simulink model "test_system_2016a"  (R2018b)
settings: Solver=VariableStepAuto  StartTime=0.0  StopTime=80  FixedStep=0.02  RelTol=1e-3  EnableMultiTasking=on
values from neighbouring files (symbols this model uses):
  c0 = g0    [init_transfers_knut.m]
  D = 50    [init_transfers_knut.m]
  FD = -X22*Y21    [init_transfers_knut.m]
  FD_f = 1    [init_transfers_knut.m]
  g0 = q0    [init_transfers_knut.m]
  H = 3.5    [init_transfers_knut.m]
  H2 = 9.6    [init_transfers_knut.m]
  hs = 1    [init_transfers_knut.m]
  K11 = 2*pi*f0*S_base/M1*bd1*(1-bd1*X22(1,1))    [init_transfers_knut.m]
  K12 = 2*pi*f0*S_base/M1*bd1*bd2*X22(1,2)    [init_transfers_knut.m]
  K13 = S_base/M1*bd1*X22(1,3)    [init_transfers_knut.m]
  K21 = 2*pi*f0*S_base/M2*bd1*bd2*X22(2,1)    [init_transfers_knut.m]
  K22 = 2*pi*f0*S_base/M2*bd2*(1-bd2*X22(2,2))    [init_transfers_knut.m]
  K23 = S_base/M2*bd2*X22(2,3)    [init_transfers_knut.m]
  Kd = 0.5    [init_transfers_knut.m]
  Kd2 = 0.1    [init_transfers_knut.m]
  Kp = 10    [init_transfers_knut.m]
  Pm0 = 0.8    [init_transfers_knut.m]
  q0 = (Pm0+(At*qnl))/(At-(w0*Dt))    [init_transfers_knut.m]
  R = 0.08    [init_transfers_knut.m]
  R2 = R    (= 0.08)    [init_transfers_knut.m]
  Td = 0    [init_transfers_knut.m]
  Tf = 0.05    [init_transfers_knut.m]
  Ti = 9.1    [init_transfers_knut.m]
  w0 = 0    [init_transfers_knut.m]
  w_ref = w0+g0*R    [init_transfers_knut.m]
undefined symbols (not defined in the file or in its folder): At, Dt, Gmax, Gmin, qnl, r, Tg, Tr, Tw
settings Model: Creator=sigurdj  LastModifiedBy=sigurd
settings DataIOCC: LimitDataPoints=on  SaveFormat=Array
settings OptimizationCC: LifeSpan=inf
settings DebuggingCC: SolverPrmCheckMsg=warning  SFUnexpectedBacktrackingDiag=warning  SFNoUnconditionalDefaultTransitionDiag=warning
settings HardwareCC: ProdBitPerPointer=32  ProdBitPerSizeT=32  ProdBitPerPtrDiffT=32  ProdLargestAtomicFloat=None  ProdIntDivRoundTo=Undefined  ProdEndianess=Unspecified  ProdWordSize=32  ProdHWDeviceType=32-bit Generic
settings ModelReferenceCC: PropagateSignalLabelsOutOfModel=off
settings SFSimCC: SimUseLocalCustomCode=off
settings RTWCC: RTWUseLocalCustomCode=off
settings CodeAppCC: StateflowObjectComments=on
settings GRTTargetCC: TargetLangStandard=C89/C90 (ANSI)  GeneratePreprocessorConditionals=Disable all
settings ConfigComp: CovMetricSettings=dw  CovHtmlReporting=on  CovSaveCumulativeToWorkspaceVar=on  CovSaveSingleToWorkspaceVar=on  CovExternalEMLEnable=off  CovSFcnEnable=off

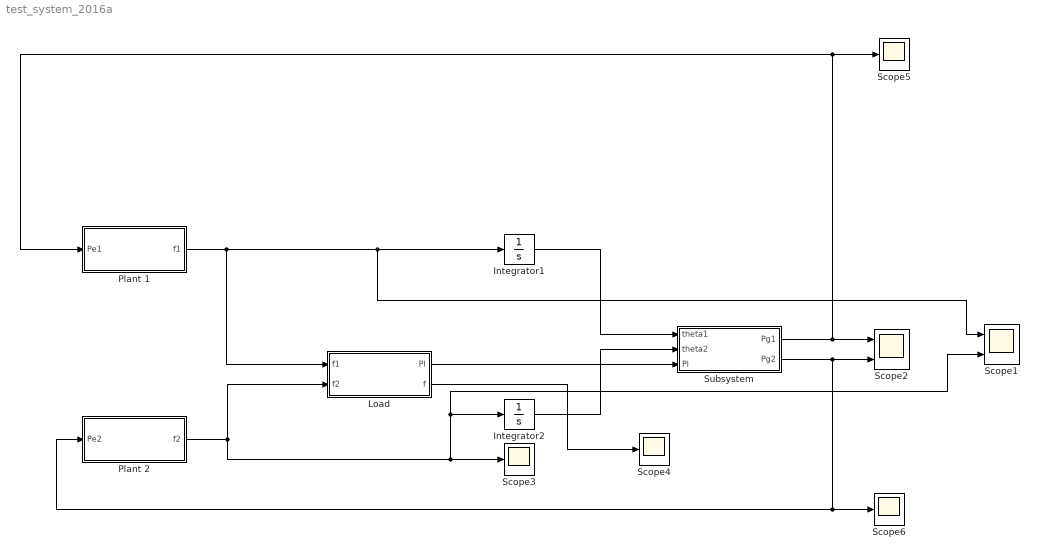
== system test_system_2016a ==
  Integrator1 : Integrator
  Integrator2 : Integrator
  Load : Subsystem
  Plant 1 : Subsystem
  Plant 2 : Subsystem
  Scope1 : Scope  NumInputPorts=2
  Scope2 : Scope  NumInputPorts=2
  Scope{3..6} (4 alike) : Scope
  Subsystem : Subsystem
  wires:
  Integrator2/1 -> Subsystem/2(theta2)
  Subsystem/2(Pg2) -> Scope2/2, Plant 2/1(Pe2), Scope6/1
  Plant 1/1(f1) -> Integrator1/1, Scope1/1, Load/1(f1)
  Plant 2/1(f2) -> Load/2(f2), Integrator2/1, Scope1/2, Scope3/1
  Integrator1/1 -> Subsystem/1(theta1)
  Subsystem/1(Pg1) -> Plant 1/1(Pe1), Scope5/1, Scope2/1
  Load/1(Pl) -> Subsystem/3(Pl)
  Load/2(f) -> Scope4/1

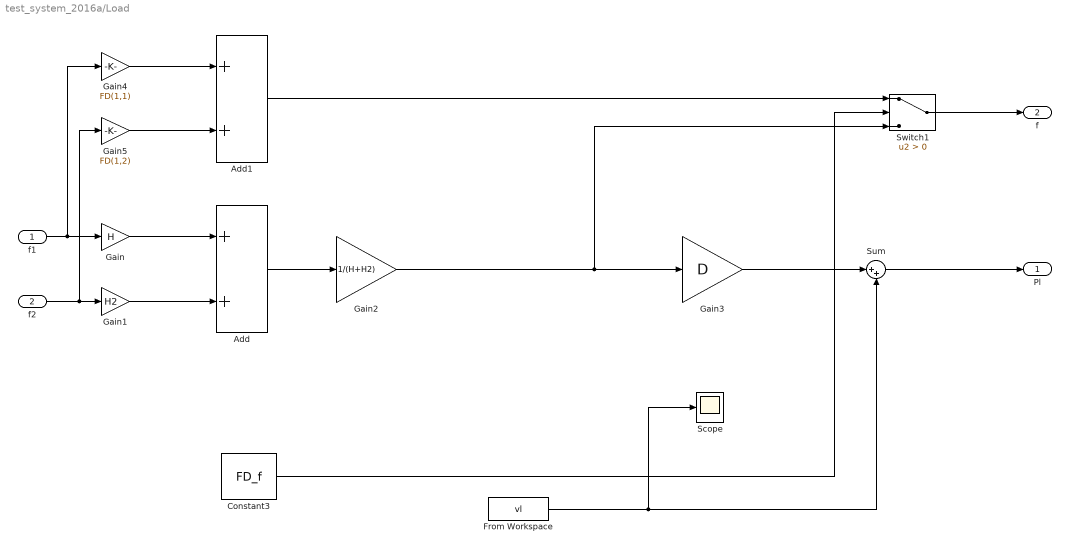
== system test_system_2016a/Load ==
  f1 : Inport
  f2 : Inport  Port=2
  Add : Sum
  Add1 : Sum
  Constant3 : Constant  Value=FD_f
  From Workspace : FromWorkspace  VariableName=vl  SampleTime=0
  Gain : Gain  Gain=H
  Gain1 : Gain  Gain=H2
  Gain2 : Gain  Gain=1/(H+H2)
  Gain3 : Gain  Gain=D
  Gain4 : Gain  Gain=FD(1,1)
  Gain5 : Gain  Gain=FD(1,2)
  Scope : Scope
  Sum : Sum  Inputs=|++
  Switch1 : Switch  Criteria=u2 > Threshold
  Pl : Outport
  f : Outport  Port=2
  wires:
  f2/1 -> Gain5/1, Gain1/1
  Gain/1 -> Add/1
  Gain1/1 -> Add/2
  Add/1 -> Gain2/1
  Sum/1 -> Pl/1
  From Workspace/1 -> Scope/1, Sum/2
  Gain2/1 -> Switch1/3, Gain3/1
  Gain4/1 -> Add1/1
  Gain5/1 -> Add1/2
  Add1/1 -> Switch1/1
  f1/1 -> Gain4/1, Gain/1
  Constant3/1 -> Switch1/2
  Switch1/1 -> f/1
  Gain3/1 -> Sum/1

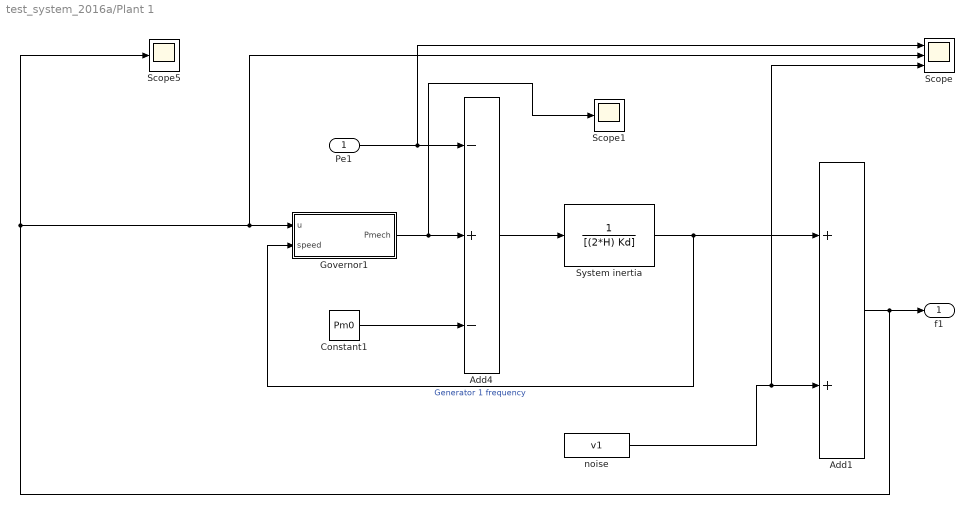
== system test_system_2016a/Plant 1 ==
  Pe1 : Inport
  Add1 : Sum
  Add4 : Sum  Inputs=-+-
  Constant1 : Constant  Value=Pm0
  Governor1 : Subsystem
  Scope : Scope  NumInputPorts=3
  Scope1 : Scope
  Scope5 : Scope
  System inertia : TransferFcn  Denominator=[(2*H) Kd]
  noise : FromWorkspace  VariableName=v1  SampleTime=0
  f1 : Outport
  wires:
  Add4/1 -> System inertia/1
  Governor1/1(Pmech) -> Scope1/1, Add4/2
  Pe1/1 -> Scope/1, Add4/1
  System inertia/1 -> Governor1/2(speed), Add1/1  "Generator 1 frequency"
  Constant1/1 -> Add4/3
  noise/1 -> Scope/3, Add1/2
  Add1/1 -> Scope/2, Governor1/1("u "), Scope5/1, f1/1

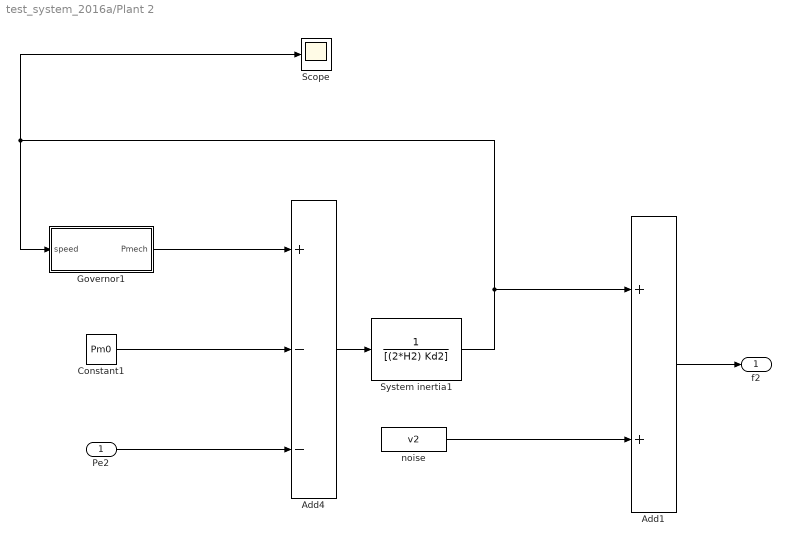
== system test_system_2016a/Plant 2 ==
  Pe2 : Inport
  Add1 : Sum
  Add4 : Sum  Inputs=+--
  Constant1 : Constant  Value=Pm0
  Governor1 : Subsystem
  Scope : Scope
  System inertia1 : TransferFcn  Denominator=[(2*H2) Kd2]
  noise : FromWorkspace  VariableName=v2  SampleTime=0
  f2 : Outport
  wires:
  System inertia1/1 -> Governor1/1(speed), Scope/1, Add1/1
  Add4/1 -> System inertia1/1
  Pe2/1 -> Add4/3
  Governor1/1(Pmech) -> Add4/1
  Constant1/1 -> Add4/2
  Add1/1 -> f2/1
  noise/1 -> Add1/2

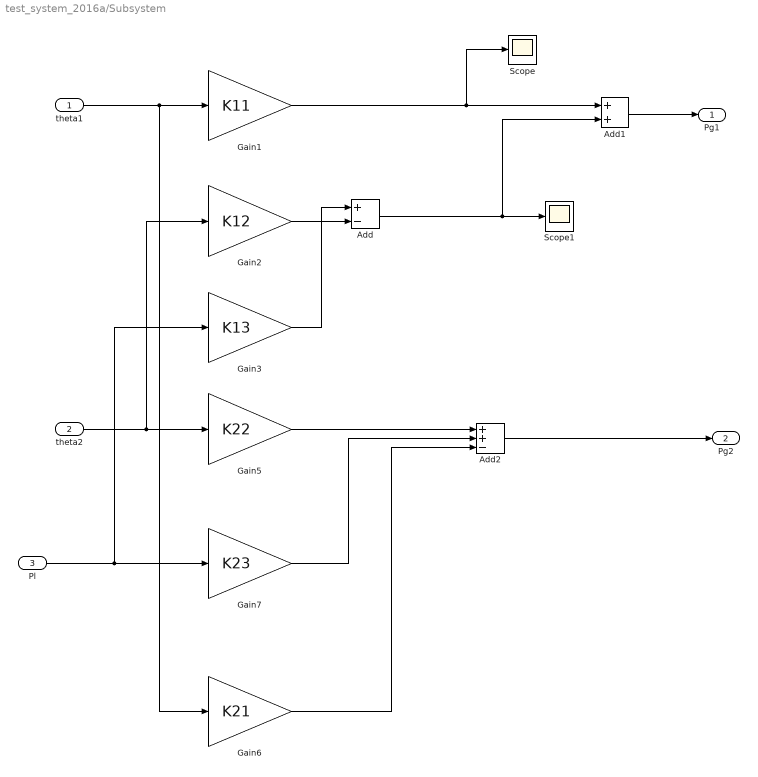
== system test_system_2016a/Subsystem ==
  theta1 : Inport  PortDimensions=1
  theta2 : Inport  Port=2  PortDimensions=1
  Pl : Inport  Port=3  PortDimensions=1
  Add : Sum  Inputs=+-
  Add1 : Sum
  Add2 : Sum  Inputs=++-
  Gain1 : Gain  Gain=K11
  Gain2 : Gain  Gain=K12
  Gain3 : Gain  Gain=K13
  Gain5 : Gain  Gain=K22
  Gain6 : Gain  Gain=K21
  Gain7 : Gain  Gain=K23
  Scope : Scope
  Scope1 : Scope
  Pg1 : Outport
  Pg2 : Outport  Port=2
  wires:
  theta1/1 -> Gain6/1, Gain1/1
  theta2/1 -> Gain5/1, Gain2/1
  Pl/1 -> Gain7/1, Gain3/1
  Gain1/1 -> Scope/1, Add1/1
  Gain3/1 -> Add/1
  Add1/1 -> Pg1/1
  Gain6/1 -> Add2/3
  Add2/1 -> Pg2/1
  Gain7/1 -> Add2/2
  Gain5/1 -> Add2/1
  Gain2/1 -> Add/2
  Add/1 -> Scope1/1, Add1/2

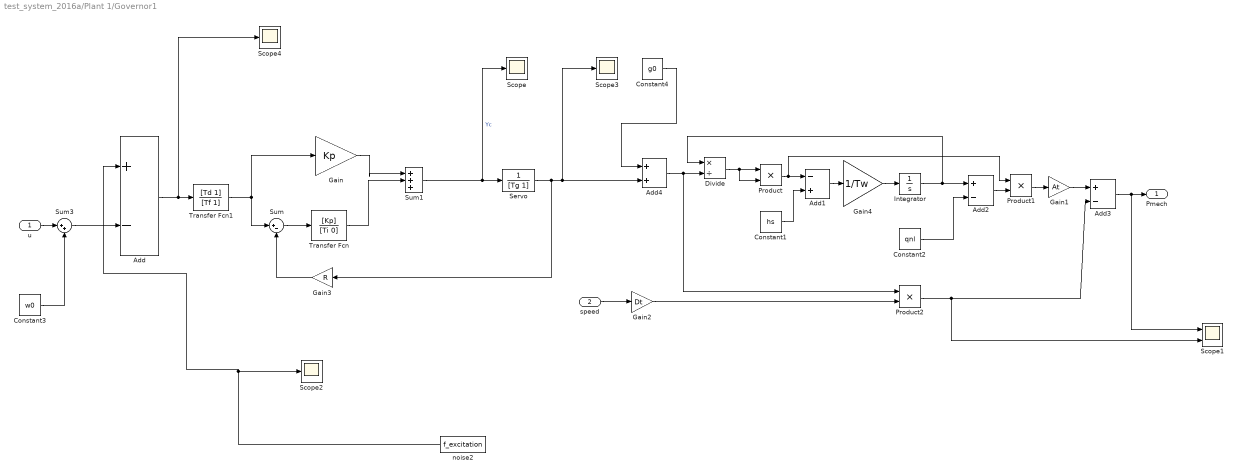
== system test_system_2016a/Plant 1/Governor1 ==
  "u " : Inport
  speed : Inport  Port=2
  Add : Sum  Inputs=+-
  Add1 : Sum  Inputs=-+
  Add2 : Sum  Inputs=+-
  Add3 : Sum  Inputs=+-
  Add4 : Sum
  Constant1 : Constant  Value=hs
  Constant2 : Constant  Value=qnl
  Constant3 : Constant  Value=w0
  Constant4 : Constant  Value=g0
  Divide : Product  Inputs=*/
  Gain : Gain  Gain=Kp
  Gain1 : Gain  Gain=At
  Gain2 : Gain  Gain=Dt
  Gain3 : Gain  Gain=R
  Gain4 : Gain  Gain=1/Tw
  Integrator : Integrator  InitialCondition=q0
  Product : Product
  Product1 : Product
  Product2 : Product
  Scope{,2..4} (4 alike) : Scope
  Scope1 : Scope  NumInputPorts=2
  Servo : TransferFcn  Denominator=[Tg 1]
  Sum : Sum  Inputs=|+-
  Sum1 : Sum  Inputs=|+++
  Sum3 : Sum  Inputs=|++
  Transfer Fcn : TransferFcn  Numerator=[Kp]  Denominator=[Ti 0]
  Transfer Fcn1 : TransferFcn  Numerator=[Td 1]  Denominator=[Tf 1]
  noise2 : FromWorkspace  VariableName=f_excitation  SampleTime=0
  Pmech : Outport
  wires:
  Divide/1 -> Product/2, Product/1
  Product2/1 -> Scope1/2, Add3/2
  Add3/1 -> Scope1/1, Pmech/1
  Gain4/1 -> Integrator/1
  Gain1/1 -> Add3/1
  Gain2/1 -> Product2/2
  Product/1 -> Product1/1, Add1/1
  Constant2/1 -> Add2/2
  Constant1/1 -> Add1/2
  Add/1 -> Scope4/1, Transfer Fcn1/1
  Product1/1 -> Gain1/1
  Add1/1 -> Gain4/1
  Integrator/1 -> Divide/1, Add2/1
  Add2/1 -> Product1/2
  "u "/1 -> Sum3/1
  Sum3/1 -> Add/2
  Constant3/1 -> Sum3/2
  speed/1 -> Gain2/1
  Constant4/1 -> Add4/1
  Add4/1 -> Product2/1, Divide/2
  Sum/1 -> Transfer Fcn/1
  Gain/1 -> Sum1/1
  Transfer Fcn/1 -> Sum1/2
  Gain3/1 -> Sum/2
  Sum1/1 -> Servo/1, Scope/1  "Yc"
  Transfer Fcn1/1 -> Sum/1, Gain/1
  Servo/1 -> Gain3/1, Scope3/1, Add4/2
  noise2/1 -> Add/1, Scope2/1

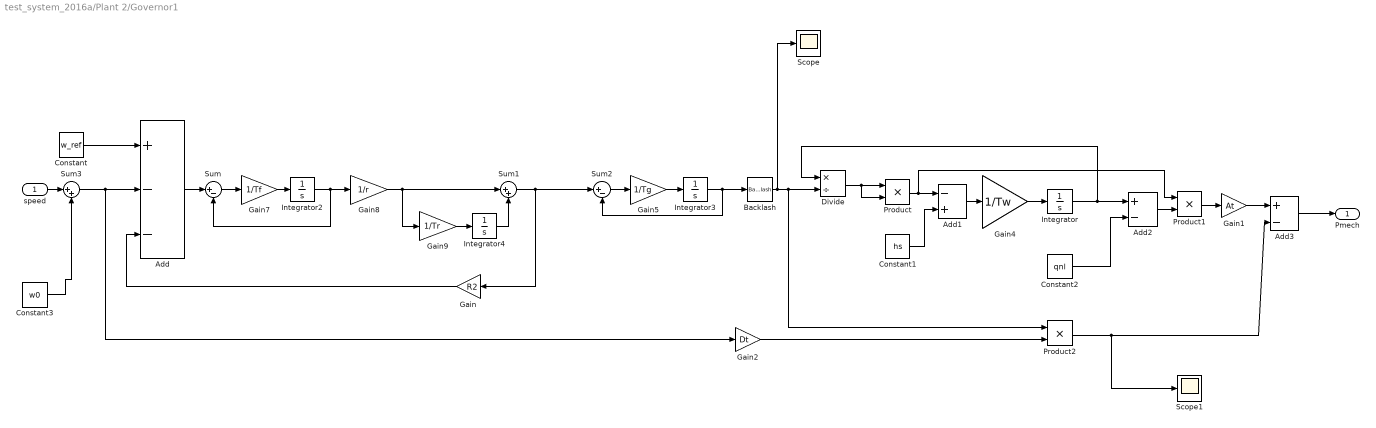
== system test_system_2016a/Plant 2/Governor1 ==
  speed : Inport
  Add : Sum  Inputs=+--
  Add1 : Sum  Inputs=-+
  Add2 : Sum  Inputs=+-
  Add3 : Sum  Inputs=+-
  Backlash : Backlash  BacklashWidth=ksp
  Constant : Constant  Value=w_ref
  Constant1 : Constant  Value=hs
  Constant2 : Constant  Value=qnl
  Constant3 : Constant  Value=w0
  Divide : Product  Inputs=*/
  Gain : Gain  Gain=R2
  Gain1 : Gain  Gain=At
  Gain2 : Gain  Gain=Dt
  Gain4 : Gain  Gain=1/Tw
  Gain5 : Gain  Gain=1/Tg
  Gain7 : Gain  Gain=1/Tf
  Gain8 : Gain  Gain=1/r
  Gain9 : Gain  Gain=1/Tr
  Integrator : Integrator  InitialCondition=q0
  Integrator2 : Integrator  UpperSaturationLimit=Gmax  LowerSaturationLimit=Gmin
  Integrator3 : Integrator  InitialCondition=g0
  Integrator4 : Integrator  InitialCondition=c0
  Product : Product
  Product1 : Product
  Product2 : Product
  Scope : Scope
  Scope1 : Scope
  Sum : Sum  Inputs=|+-
  Sum1 : Sum  Inputs=|++
  Sum2 : Sum  Inputs=|+-
  Sum3 : Sum  Inputs=|++
  Pmech : Outport
  wires:
  Gain5/1 -> Integrator3/1
  Integrator4/1 -> Sum1/2
  Gain7/1 -> Integrator2/1
  Sum/1 -> Gain7/1
  Divide/1 -> Product/2, Product/1
  Product2/1 -> Scope1/1, Add3/2
  Add3/1 -> Pmech/1
  Gain4/1 -> Integrator/1
  Gain8/1 -> Sum1/1, Gain9/1
  Gain1/1 -> Add3/1
  Gain2/1 -> Product2/2
  Product/1 -> Product1/1, Add1/1
  Constant2/1 -> Add2/2
  Gain/1 -> Add/3
  Constant1/1 -> Add1/2
  Add/1 -> Sum/1
  Product1/1 -> Gain1/1
  Constant/1 -> Add/1
  Gain9/1 -> Integrator4/1
  Add1/1 -> Gain4/1
  Sum2/1 -> Gain5/1
  Integrator2/1 -> Gain8/1, Sum/2
  Integrator/1 -> Divide/1, Add2/1
  Add2/1 -> Product1/2
  Backlash/1 -> Scope/1, Divide/2, Product2/1
  Integrator3/1 -> Backlash/1, Sum2/2
  speed/1 -> Sum3/1
  Sum3/1 -> Add/2, Gain2/1
  Constant3/1 -> Sum3/2
  Sum1/1 -> Sum2/1, Gain/1
